simulink model "AccTarSel"  (R2018b)
settings: Solver=FixedStepDiscrete  StartTime=0.0  StopTime=inf  FixedStep=0.01  RelTol=1e-3
PostLoadFcn:
  | if any(exist('dsrtsu_mdlpostloadfcn', 'file') ~= 0), dsrtsu_mdlpostloadfcn('Execute', bdroot); end
values from neighbouring files (symbols this model uses):
  P_adtMaxBDC = 1.0    [AccTarSel.sldd]
  P_aFOCApproachIntpAcitve = -0.6    [AccTarSel.sldd]
  P_aFOCApproachIntpEnsure = -1.8    [AccTarSel.sldd]
  P_CutInEnable = 1.0    [AccTarSel.sldd]
  P_dAimMin = 4.5    [AccTarSel.sldd]
  P_dAimMinAVP = 1.5    [AccTarSel.sldd]
  P_dObjDrvOffMax = 5.0    [AccTarSel.sldd]
  P_dObjDrvOffMin = 3.0    [AccTarSel.sldd]
  P_dObjLowHystDecToStop = 4.5    [AccTarSel.sldd]
  P_dObjLowHystDecToStopAVP = 1.5    [AccTarSel.sldd]
  P_dObjUpperHystDecToStop = 5.0    [AccTarSel.sldd]
  P_dResMax = 5.0    [AccTarSel.sldd]
  P_dStandStill = 3.0    [AccTarSel.sldd]
  P_dStandStillMin = 2.0    [AccTarSel.sldd]
  P_dvarYMax4PO = 1.0    [AccTarSel.sldd]
  P_dyCutInThres = 3.6    [AccTarSel.sldd]
  P_facBDCInit = 0.7    [AccTarSel.sldd]
  P_facBDCIterCalc = 0.8    [AccTarSel.sldd]
  P_facFOCNegDiff = 0.3    [AccTarSel.sldd]
  P_facFOCPosDiff = 0.2    [AccTarSel.sldd]
  P_kapHystThres = 0.0005    [AccTarSel.sldd]
  P_PlausIntegDisable = 0.0    [AccTarSel.sldd]
  P_plausMin4PO = 0.5    [AccTarSel.sldd]
  P_probExistMin4PO = 0.8    [AccTarSel.sldd]
  P_StandObjEnable = 0.0    [AccTarSel.sldd]
  P_tAxTrackNegLower = 0.3    [AccTarSel.sldd]
  P_tAxTrackNegUpper = 0.6    [AccTarSel.sldd]
  P_tAxTrackPosLower = 1.0    [AccTarSel.sldd]
  P_tAxTrackPosUpper = 2.0    [AccTarSel.sldd]
  P_tBDCStartFilt = 0.2    [AccTarSel.sldd]
  P_tCSC = 3.5    [AccTarSel.sldd]
  P_tCurvFilt = 0.2    [AccTarSel.sldd]
  P_tCutInFilt = 0.5    [AccTarSel.sldd]
  P_tFiltAxAbsPONegFast = 0.1    [AccTarSel.sldd]
  P_tFiltAxAbsPONegSlow = 0.4    [AccTarSel.sldd]
  P_tFiltAxAbsPOPosFast = 1.2    [AccTarSel.sldd]
  P_tFiltAxAbsPOPosSlow = 2.0    [AccTarSel.sldd]
  P_tFiltAxAbsPOStand = 2.0    [AccTarSel.sldd]
  P_tFiltDAim = 0.1    [AccTarSel.sldd]
  P_tFiltDsd = 0.1    [AccTarSel.sldd]
  P_tFiltSpdLim = 3.0    [AccTarSel.sldd]
  P_tFiltVxAxPOFast = 0.15    [AccTarSel.sldd]
  P_tFiltVxAxPOSlow = 0.25    [AccTarSel.sldd]
  P_tFOCStatAccelFast = 4.0    [AccTarSel.sldd]
  P_tFOCStatAccelSlow = 3.5    [AccTarSel.sldd]
  P_tFOCStatDecelFast = 4.0    [AccTarSel.sldd]
  P_tFOCStatDecelSlow = 3.2    [AccTarSel.sldd]
  P_tMinDrvPhase = 2.0    [AccTarSel.sldd]
  P_tPredObjLeav = 1.2    [AccTarSel.sldd]
  P_tRollingFilt = 0.5    [AccTarSel.sldd]
  P_tRollingFinFilt = 1.0    [AccTarSel.sldd]
  P_tSSCNeg = 4.5    [AccTarSel.sldd]
  P_tSSCPos = 5.5    [AccTarSel.sldd]
  P_tToStop = 5.0    [AccTarSel.sldd]
  P_tToStopInBDC = 6.0    [AccTarSel.sldd]
  P_tToStopTrig = 4.0    [AccTarSel.sldd]
  P_vEgoDecToStop = 3.0    [AccTarSel.sldd]
  P_vEgoLowBDC = 4.0    [AccTarSel.sldd]
  P_vFOCNegDiff = 4.0    [AccTarSel.sldd]
  P_vFOCPosDiff = 5.0    [AccTarSel.sldd]
  P_vFOCStationaryFast = 15.0    [AccTarSel.sldd]
  P_vFOCStationarySlow = 5.0    [AccTarSel.sldd]
  P_vObjDrvOff = 0.5    [AccTarSel.sldd]
  P_vObjLowHystDecToStop = 0.5    [AccTarSel.sldd]
  P_vObjNoStop = 1.0    [AccTarSel.sldd]
  P_vObjReCalc = 1.0    [AccTarSel.sldd]
  P_vObjStop = 0.3    [AccTarSel.sldd]
  P_vObjUpperHystDecToStop = 0.8    [AccTarSel.sldd]
  P_vStandStill = 0.3    [AccTarSel.sldd]
  P_vStandStillHyst = 0.3    [AccTarSel.sldd]
  P_vyCutInThres = 0.5    [AccTarSel.sldd]
libraries: simulink x21, LPFilter x12
(part 2 of 11)

== system AccTarSel/EgoCourseFusion ==
  egoInfo : Inport
  SYS_Info_st : Inport  Port=2
  Bus Creator : BusCreator  Inputs=4  OutDataTypeStr=Bus: TRAJ_LANE_ST
  Bus Selector : BusSelector  OutputSignals=Curvature
  Bus Selector1 : BusSelector  OutputSignals=dT
  Constant2 : Constant  Value=0.5  OutDataTypeStr=single
  Constant3 : Constant  Value=0  OutDataTypeStr=single
  Constant4 : Constant  Value=0  OutDataTypeStr=single
  Constant5 : Constant  Value=0  OutDataTypeStr=single
  CurvatureFilt : Subsystem
  Multiply : Product
  egoTrajLane_st : Outport
  wires:
  Bus Creator/1 -> egoTrajLane_st/1  "egoTrajLane_st"
  CurvatureFilt/1(kapTrajFilt) -> Multiply/1  "kapTrajFilt"
  Constant2/1 -> Multiply/2
  Constant4/1 -> Bus Creator/3  "c"
  Constant3/1 -> Bus Creator/1  "a"
  Multiply/1 -> Bus Creator/2  "b"
  Constant5/1 -> Bus Creator/4  "d"
  egoInfo/1 -> Bus Selector/1
  Bus Selector/1 -> CurvatureFilt/1(In1)  "<Curvature>"
  SYS_Info_st/1 -> Bus Selector1/1
  Bus Selector1/1 -> CurvatureFilt/2(In2)  "<dT>"

== system AccTarSel/ObjAdapter ==
  FusObjIn : Inport
  egoInfo : Inport  Port=2
  Bus Creator : BusCreator  Inputs=2  OutDataTypeStr=Bus: FUS_OBJDATA_ST  NonVirtualBus=on
  Bus Selector : BusSelector  OutputSignals=objects
  Constant : Constant  Value=0  OutDataTypeStr=double
  For Each Subsystem : Subsystem  TreatAsAtomicUnit=on
  FusObjOut : Outport  OutDataTypeStr=Bus: FUS_OBJDATA_ST
  wires:
  FusObjIn/1 -> Bus Selector/1
  Bus Selector/1 -> For Each Subsystem/1(In1)  "<objects>"
  Bus Creator/1 -> FusObjOut/1
  For Each Subsystem/1(Out1) -> Bus Creator/2  "objdata_st"
  Constant/1 -> Bus Creator/1  "timeStamp"
  egoInfo/1 -> For Each Subsystem/2(In2)

== system AccTarSel/ObjRadarAdapter ==
  In1 : Inport
  Bus Creator : BusCreator  Inputs=2  OutDataTypeStr=Bus: FUS_OBJDATA_ST  NonVirtualBus=on
      settings: InheritFromInputs=off
  Bus Selector : BusSelector  OutputSignals=x50_20_Obj_00,x51_21_Obj_01,x52_22_Obj_02,x53_23_Obj_03,x54_24_Obj_04,x55_25_Obj_05,x56_26_Obj_06,x57_27_Obj_07,x58_28_Obj_08,x59_29_Obj_09,x5A_2A_Obj_10,x5B_2B_Obj_11,x5C_2C_Obj_12,x5D_2D_Obj_13,x5E_2E_Obj_14,x5F_2F_Obj_15,x60_30_Obj_16,x61_31_Obj_17,x62_32_Obj_18,x63_33_Obj_19,x64_34_Obj_20,x65_35_Obj_21,x66_36_Obj_22,x67_37_Obj_23,x68_38_Obj_24,x69_39_Obj_25,x6A_3A_Obj_26,x6B_3B_Obj_27,x6C_3C_Obj_28,x6D_3D_Obj_29,x6E_3E_Obj_30,x6F_3F_Obj_31,x70_40_Obj_32,x71_41_Obj_33,x72_42_Obj_34,x73_43_Obj_35,x74_44_Obj_36,x75_45_Obj_37,x76_46_Obj_38,x77_47_Obj_39
  Constant : Constant  Value=0  OutDataTypeStr=double
  For Each Subsystem : Subsystem  TreatAsAtomicUnit=on
  Vector Concatenate : Concatenate  NumInputs=40
  RadarObjOut : Outport  OutDataTypeStr=Bus: FUS_OBJDATA_ST
  wires:
  In1/1 -> Bus Selector/1
  Bus Selector/1 -> Vector Concatenate/1  "<x50_20_Obj_00>"
  Bus Selector/2 -> Vector Concatenate/2  "<x51_21_Obj_01>"
  Bus Selector/3 -> Vector Concatenate/3  "<x52_22_Obj_02>"
  Bus Selector/4 -> Vector Concatenate/4  "<x53_23_Obj_03>"
  Bus Selector/5 -> Vector Concatenate/5  "<x54_24_Obj_04>"
  Bus Selector/6 -> Vector Concatenate/6  "<x55_25_Obj_05>"
  Bus Selector/7 -> Vector Concatenate/7  "<x56_26_Obj_06>"
  Bus Selector/8 -> Vector Concatenate/8  "<x57_27_Obj_07>"
  Bus Selector/9 -> Vector Concatenate/9  "<x58_28_Obj_08>"
  Bus Selector/10 -> Vector Concatenate/10  "<x59_29_Obj_09>"
  Bus Selector/11 -> Vector Concatenate/11  "<x5A_2A_Obj_10>"
  Bus Selector/12 -> Vector Concatenate/12  "<x5B_2B_Obj_11>"
  Bus Selector/13 -> Vector Concatenate/13  "<x5C_2C_Obj_12>"
  Bus Selector/14 -> Vector Concatenate/14  "<x5D_2D_Obj_13>"
  Bus Selector/15 -> Vector Concatenate/15  "<x5E_2E_Obj_14>"
  Bus Selector/16 -> Vector Concatenate/16  "<x5F_2F_Obj_15>"
  Bus Selector/17 -> Vector Concatenate/17  "<x60_30_Obj_16>"
  Bus Selector/18 -> Vector Concatenate/18  "<x61_31_Obj_17>"
  Bus Selector/19 -> Vector Concatenate/19  "<x62_32_Obj_18>"
  Bus Selector/20 -> Vector Concatenate/20  "<x63_33_Obj_19>"
  Bus Selector/21 -> Vector Concatenate/21  "<x64_34_Obj_20>"
  Bus Selector/22 -> Vector Concatenate/22  "<x65_35_Obj_21>"
  Bus Selector/23 -> Vector Concatenate/23  "<x66_36_Obj_22>"
  Bus Selector/24 -> Vector Concatenate/24  "<x67_37_Obj_23>"
  Bus Selector/25 -> Vector Concatenate/25  "<x68_38_Obj_24>"
  Bus Selector/26 -> Vector Concatenate/26  "<x69_39_Obj_25>"
  Bus Selector/27 -> Vector Concatenate/27  "<x6A_3A_Obj_26>"
  Bus Selector/28 -> Vector Concatenate/28  "<x6B_3B_Obj_27>"
  Bus Selector/29 -> Vector Concatenate/29  "<x6C_3C_Obj_28>"
  Bus Selector/30 -> Vector Concatenate/30  "<x6D_3D_Obj_29>"
  Bus Selector/31 -> Vector Concatenate/31  "<x6E_3E_Obj_30>"
  Bus Selector/32 -> Vector Concatenate/32  "<x6F_3F_Obj_31>"
  Bus Selector/33 -> Vector Concatenate/33  "<x70_40_Obj_32>"
  Bus Selector/34 -> Vector Concatenate/34  "<x71_41_Obj_33>"
  Bus Selector/35 -> Vector Concatenate/35  "<x72_42_Obj_34>"
  Bus Selector/36 -> Vector Concatenate/36  "<x73_43_Obj_35>"
  Bus Selector/37 -> Vector Concatenate/37  "<x74_44_Obj_36>"
  Bus Selector/38 -> Vector Concatenate/38  "<x75_45_Obj_37>"
  Bus Selector/39 -> Vector Concatenate/39  "<x76_46_Obj_38>"
  Bus Selector/40 -> Vector Concatenate/40  "<x77_47_Obj_39>"
  Vector Concatenate/1 -> For Each Subsystem/1(In1)
  For Each Subsystem/1(Out1) -> Bus Creator/2  "objdata_st"
  Bus Creator/1 -> RadarObjOut/1
  Constant/1 -> Bus Creator/1  "timeStamp"

== system AccTarSel/RTI Data ==
  RTI Data Store : Subsystem  Tag="struct('private',struct('version',struct('dsVer',uint32(2),'dsVerCreation',uint32(2),'RTI',struct('ver','7.12','type','RTI1401')),'access',struct('type','Model','isPerm',1,'created',['19-Nov-2020 15:49:14'],'modified',['12-Mar-2021 13:34:18'],'location','')),'public',struct('main',struct('data',[]),'sub',struct('name',{{'AccTarSel'}},'data',{{struct('TH',struct('thTaskInfo',struct('taskType',{'TIMER','HWINT','TMRINT','SWINT','GLINT'},'tasksNumOf',{1,0,0,0,0},'srcIds',{{'TIMERA'},{},{},{},{}},'taskNames',{{['Timer Task 1']},{},{},{},{}})),'th_tc',struct('dataType','TASK','taskGroupId','','taskGroupList',{{}},'taskSchedulingPolicy','FCFS','taskType','TIMER','blkh',-1,'srcId','TIMERA','srcSgnName',['Timer A interrupt'],'srcCpuName','','taskName',['Timer Task 1  [0.005] s'],'taskNameDisplayExt','','smplTime',0.005,'smplTimeOffs',0,'hasFixedPriority',0,'priority',1,'hasFixedOvc',0,'ovcType',1,'ovcMax',1),'tc_th',struct('dataType','TASK','taskGroupId','','taskGroupList',{{}},'taskSchedulingPolicy','FCFS','taskType','TIMER','blkh',-1,'srcId','TIMERA','srcSgnName',['Timer A interrupt'],'srcCpuName','','taskName',['Timer Task 1  [0.005] s'],'taskNameDisplayExt','','smplTime',0.005,'smplTimeOffs',0,'hasFixedPriority',0,'priority',1,'hasFixedOvc',0,'ovcType',1,'ovcMax',1))}})))"  mask(RTI_DATA_STORE){}
      mask help:
      | RTI Data Store Block. This block is used by RTI to store internal model dependent data. Deleting this block will result in data loss.
      |
      | NEVER DELETE, COPY, OR MODIFY THIS BLOCK!
      mask Help:
      | RTI Data Store Block. This block is used by RTI to store internal model dependent data. Deleting this block will result in data loss.
      | 
      | NEVER DELETE, COPY, OR MODIFY THIS BLOCK!
      mask Display: text(0.5, 0.5, ' ', 'HorizontalAlignment', 'center');

== system AccTarSel/Subsystem ==
  In1 : Inport
  In2 : Inport  Port=2
  Bus Creator : BusCreator  Inputs=2  OutDataTypeStr=Bus: FUS_OBJDATA_ST  NonVirtualBus=on
  Bus Selector : BusSelector  OutputSignals=timeStamp,objdata_st
  Bus Selector1 : BusSelector  OutputSignals=objdata_st
  Vector Concatenate : Concatenate  ConcatenateDimension=2
  Out1 : Outport
  wires:
  In1/1 -> Bus Selector/1
  In2/1 -> Bus Selector1/1
  Bus Selector1/1 -> Vector Concatenate/2  "<objdata_st>"
  Bus Selector/2 -> Vector Concatenate/1  "<objdata_st>"
  Bus Selector/1 -> Bus Creator/1  "<timeStamp>"
  Vector Concatenate/1 -> Bus Creator/2  "objdata_st"
  Bus Creator/1 -> Out1/1

== system AccTarSel/Subsystem1 ==
  objInfo : Inport
  egoInfo : Inport  Port=2
  AND2 : Logic  AllPortsSameDT=off  OutDataTypeStr=boolean
  AND3 : Logic  Operator=OR  AllPortsSameDT=off  OutDataTypeStr=boolean
  Add : Sum
  Bus Selector : BusSelector  OutputSignals=Valid,dx,vx
  Bus Selector1 : BusSelector  OutputSignals=vRef
  Constant : Constant  OutDataTypeStr=boolean
  Constant1 : Constant  Value=0  OutDataTypeStr=int32
  If : If  IfExpression=u1 == 1
  If Action Subsystem : Subsystem  TreatAsAtomicUnit=on
  If Action Subsystem1 : Subsystem  TreatAsAtomicUnit=on
  Merge : Merge
  P_dObjDrvOffMax : Constant  Value=P_dObjDrvOffMax
  P_dObjDrvOffMin : Constant  Value=P_dObjDrvOffMin
  P_vObjDrvOff : Constant  Value=P_vObjDrvOff
  Relational Operator6 : RelationalOperator  Operator=>  OutDataTypeStr=boolean  RndMeth=Simplest
  Relational Operator7 : RelationalOperator  Operator=>  OutDataTypeStr=boolean  RndMeth=Simplest
  Relational Operator8 : RelationalOperator  Operator=>  OutDataTypeStr=boolean  RndMeth=Simplest
  Selector1 : Selector  IndexMode=Zero-based  InputPortWidth=6  IndexOptions=Index vector (port)  Indices=[1 3]  OutputSizes=1
  DrvOffEnable : Outport
  wires:
  AND2/1 -> AND3/2
  Relational Operator8/1 -> AND2/2
  Add/1 -> Relational Operator8/1  "vAbsObj"
  P_dObjDrvOffMin/1 -> Relational Operator7/2
  Relational Operator7/1 -> AND2/1
  Relational Operator6/1 -> AND3/1
  P_vObjDrvOff/1 -> Relational Operator8/2
  P_dObjDrvOffMax/1 -> Relational Operator6/2
  Bus Selector/1 -> If/1  "<Valid>"
  egoInfo/1 -> Bus Selector1/1
  Bus Selector1/1 -> Add/2  "<vRef>"
  Bus Selector/3 -> Add/1  "<vx>"
  Bus Selector/2 -> Relational Operator6/1, Relational Operator7/1  "<dx>"
  AND3/1 -> If Action Subsystem/1(In1)
  Constant/1 -> If Action Subsystem1/1(In1)
  If/1 -> If Action Subsystem/Action
  If/2 -> If Action Subsystem1/Action
  If Action Subsystem/1(Out1) -> Merge/1
  If Action Subsystem1/1(Out1) -> Merge/2
  Merge/1 -> DrvOffEnable/1  "DrvOffEnable"
  objInfo/1 -> Selector1/1
  Constant1/1 -> Selector1/2
  Selector1/1 -> Bus Selector/1

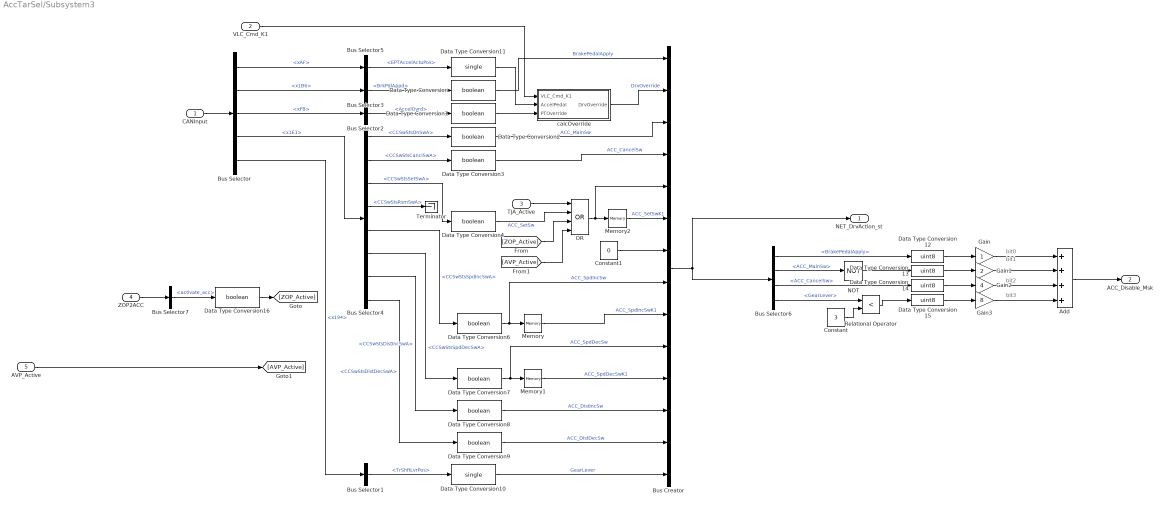
== system AccTarSel/Subsystem3 ==
  note: bit0
  note: bit1
  note: bit2
  note: bit3
  CANInput : Inport
  VLC_Cmd_K1 : Inport  Port=2
  TJA_Active : Inport  Port=3
  ZOP2ACC : Inport  Port=4
  AVP_Active : Inport  Port=5
  Add : Sum  Inputs=++++  AccumDataTypeStr=uint16
  Bus Creator : BusCreator  Inputs=14  OutDataTypeStr=Bus: NET_DRVACTION_ST  NonVirtualBus=on
      settings: InheritFromInputs=off
  Bus Selector : BusSelector  OutputSignals=xAF,x1B6,xFB,x1E1,x194
  Bus Selector1 : BusSelector  OutputSignals=TrShftLvrPos
  Bus Selector2 : BusSelector  OutputSignals=AccelOvrd
  Bus Selector3 : BusSelector  OutputSignals=BrkPdlAppd
  Bus Selector4 : BusSelector  OutputSignals=CCSwStsOnSwA,CCSwStsCanclSwA,CCSwStsSetSwA,CCSwStsRsmSwA,CCSwStsSpdIncSwA,CCSwStsSpdDecSwA,CCSwStsDistIncSwA,CCSwStsDistDecSwA
  Bus Selector5 : BusSelector  OutputSignals=EPTAccelActuPos
  Bus Selector6 : BusSelector  OutputSignals=BrakePedalApply,ACC_MainSw,ACC_CancelSw,GearLever
  Bus Selector7 : BusSelector  OutputSignals=activate_acc
  Constant : Constant  Value=3  OutDataTypeStr=single
  Constant1 : Constant  Value=0  OutDataTypeStr=boolean
  Data Type Conversion{,1..4,6..9,16} (10 alike) : DataTypeConversion  OutDataTypeStr=boolean
  Data Type Conversion10 : DataTypeConversion  OutDataTypeStr=single
  Data Type Conversion11 : DataTypeConversion  OutDataTypeStr=single
  Data Type Conversion{12..15} (4 alike) : DataTypeConversion  OutDataTypeStr=uint8
  Gain : Gain  OutDataTypeStr=uint16
  Gain1 : Gain  Gain=2  OutDataTypeStr=uint16
  Gain2 : Gain  Gain=4  OutDataTypeStr=uint16
  Gain3 : Gain  Gain=8  OutDataTypeStr=uint16
  Memory : Memory
  Memory1 : Memory
  Memory2 : Memory
  NOT : Logic  Operator=NOT  AllPortsSameDT=off  OutDataTypeStr=boolean
  OR : Logic  Operator=OR  Inputs=4  AllPortsSameDT=off  OutDataTypeStr=boolean
  Relational Operator : RelationalOperator  Operator=<  OutDataTypeStr=boolean  RndMeth=Simplest
  Terminator : Terminator
  calcOverride : Subsystem
  NET_DrvAction_st : Outport  OutDataTypeStr=Bus: NET_DRVACTION_ST
  ACC_Disable_Msk : Outport  Port=2
  wires:
  CANInput/1 -> Bus Selector/1
  Bus Selector/5 -> Bus Selector1/1  "<x194>"
  Bus Selector/3 -> Bus Selector2/1  "<xFB>"
  Bus Selector/2 -> Bus Selector3/1  "<x1B6>"
  Bus Selector/4 -> Bus Selector4/1  "<x1E1>"
  Bus Selector3/1 -> Data Type Conversion/1  "<BrkPdlAppd>"
  Data Type Conversion/1 -> Bus Creator/1  "BrakePedalApply"
  Bus Selector2/1 -> Data Type Conversion1/1  "<AccelOvrd>"
  Bus Selector4/1 -> Data Type Conversion2/1  "<CCSwStsOnSwA>"
  Bus Selector4/2 -> Data Type Conversion3/1  "<CCSwStsCanclSwA>"
  Bus Selector4/3 -> Data Type Conversion4/1  "<CCSwStsSetSwA>"
  Bus Selector4/4 -> Terminator/1  "<CCSwStsRsmSwA>"
  Bus Selector4/5 -> Data Type Conversion6/1  "<CCSwStsSpdIncSwA>"
  Bus Selector4/6 -> Data Type Conversion7/1  "<CCSwStsSpdDecSwA>"
  Data Type Conversion6/1 -> Bus Creator/8, Memory/1  "ACC_SpdIncSw"
  Memory/1 -> Bus Creator/9  "ACC_SpdIncSwK1"
  Data Type Conversion7/1 -> Bus Creator/10, Memory1/1  "ACC_SpdDecSw"
  Memory1/1 -> Bus Creator/11  "ACC_SpdDecSwK1"
  Data Type Conversion8/1 -> Bus Creator/12  "ACC_DistIncSw"
  Bus Selector4/7 -> Data Type Conversion8/1  "<CCSwStsDistIncSwA>"
  Data Type Conversion9/1 -> Bus Creator/13  "ACC_DistDecSw"
  Bus Selector4/8 -> Data Type Conversion9/1  "<CCSwStsDistDecSwA>"
  Data Type Conversion2/1 -> Bus Creator/3  "ACC_MainSw"
  Data Type Conversion3/1 -> Bus Creator/4  "ACC_CancelSw"
  Bus Creator/1 -> NET_DrvAction_st/1, Bus Selector6/1
  Data Type Conversion10/1 -> Bus Creator/14  "GearLever"
  Bus Selector1/1 -> Data Type Conversion10/1  "<TrShftLvrPos>"
  Bus Selector/1 -> Bus Selector5/1  "<xAF>"
  Bus Selector5/1 -> Data Type Conversion11/1  "<EPTAccelActuPos>"
  calcOverride/1(DrvOverride) -> Bus Creator/2  "DrvOverride"
  VLC_Cmd_K1/1 -> calcOverride/1(VLC_Cmd_K1)
  Data Type Conversion11/1 -> calcOverride/2(AccelPedal)
  Data Type Conversion1/1 -> calcOverride/3(PTOverride)
  Memory2/1 -> Bus Creator/6  "ACC_SetSwK1"
  Bus Selector6/1 -> Data Type Conversion12/1  "<BrakePedalApply>"
  Bus Selector6/3 -> Data Type Conversion14/1  "<ACC_CancelSw>"
  Bus Selector6/2 -> NOT/1  "<ACC_MainSw>"
  NOT/1 -> Data Type Conversion13/1
  Bus Selector6/4 -> Relational Operator/1  "<GearLever>"
  Constant/1 -> Relational Operator/2
  Relational Operator/1 -> Data Type Conversion15/1
  Data Type Conversion12/1 -> Gain/1
  Data Type Conversion13/1 -> Gain1/1
  Data Type Conversion14/1 -> Gain2/1
  Data Type Conversion15/1 -> Gain3/1
  Gain/1 -> Add/1
  Gain1/1 -> Add/2
  Gain2/1 -> Add/3
  Gain3/1 -> Add/4
  Add/1 -> ACC_Disable_Msk/1
  TJA_Active/1 -> OR/1
  Data Type Conversion4/1 -> OR/2  "ACC_SetSw"
  OR/1 -> Bus Creator/5, Memory2/1
  Constant1/1 -> Bus Creator/7
  ZOP2ACC/1 -> Bus Selector7/1
  Bus Selector7/1 -> Data Type Conversion16/1  "<activate_acc>"
  Data Type Conversion16/1 -> [ZOP_Active]
  [ZOP_Active] -> OR/3
  AVP_Active/1 -> [AVP_Active]
  [AVP_Active] -> OR/4

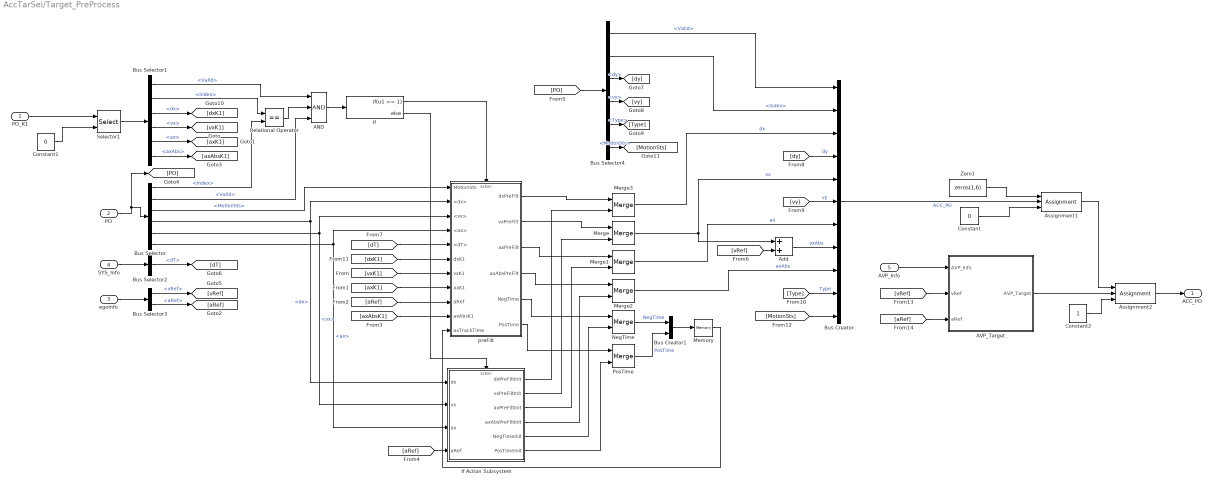
== system AccTarSel/Target_PreProcess ==
  PO_K1 : Inport
  PO : Inport  Port=2
  egoInfo : Inport  Port=3
  SYS_Info : Inport  Port=4
  AVP_Info : Inport  Port=5
  AND : Logic  Inputs=3  AllPortsSameDT=off  OutDataTypeStr=boolean
  AVP_Target : Subsystem
  Add : Sum
  Assignment1 : Assignment  IndexMode=Zero-based  DiagnosticForDimensions=Warning  IndexOptions=Index vector (port)  Indices=1  OutputSizes=1
  Assignment2 : Assignment  IndexMode=Zero-based  DiagnosticForDimensions=Warning  IndexOptions=Index vector (port)  Indices=1  OutputSizes=1
  Bus Creator : BusCreator  Inputs=11  OutDataTypeStr=Bus: ATS_PO_ST  NonVirtualBus=on
      settings: InheritFromInputs=off
  Bus Creator1 : BusCreator  Inputs=2
  Bus Selector : BusSelector  OutputSignals=Index,Valid,MotionSts,dx,vx,ax
  Bus Selector1 : BusSelector  OutputSignals=Valid,Index,dx,vx,ax,axAbs
  Bus Selector2 : BusSelector  OutputSignals=dT
  Bus Selector3 : BusSelector  OutputSignals=vRef,aRef
  Bus Selector4 : BusSelector  OutputSignals=Valid,Index,dy,vy,Type,MotionSts
  Constant : Constant  Value=0  OutDataTypeStr=int32
  Constant1 : Constant  Value=0  OutDataTypeStr=int32
  Constant2 : Constant  OutDataTypeStr=int32
  If : If  IfExpression=u1 == 1
  If Action Subsystem : Subsystem  TreatAsAtomicUnit=on
  Memory : Memory
  Merge{,1..3} (4 alike) : Merge
  NegTime : Merge
  PosTime : Merge
  Relational Operator : RelationalOperator  Operator===  OutDataTypeStr=boolean  RndMeth=Simplest
  Selector1 : Selector  IndexMode=Zero-based  InputPortWidth=6  IndexOptions=Index vector (port)  Indices=[1 3]  OutputSizes=1
  Zero1 : Constant  Value=zeros(1,6)  OutDataTypeStr=Bus: ATS_PO_ST
  preFilt : Subsystem
  ACC_PO : Outport  OutDataTypeStr=Bus: ATS_PO_ST
  wires:
  PO/1 -> [PO], Bus Selector/1
  Bus Selector1/1 -> AND/1  "<Valid>"
  Bus Selector1/2 -> Relational Operator/1  "<Index>"
  Bus Selector/1 -> Relational Operator/2  "<Index>"
  Relational Operator/1 -> AND/2
  Bus Selector/2 -> AND/3  "<Valid>"
  SYS_Info/1 -> Bus Selector2/1
  Bus Selector1/4 -> [vxK1]  "<vx>"
  Bus Selector1/5 -> [axK1]  "<ax>"
  AND/1 -> If/1
  Bus Selector/5 -> preFilt/3(<vx>), If Action Subsystem/2(vx)  "<vx>"
  Bus Selector/6 -> preFilt/4(<ax>), If Action Subsystem/3(ax)  "<ax>"
  [vxK1] -> preFilt/7(vxK1)
  [axK1] -> preFilt/8(axK1)
  If/1 -> preFilt/Action
  If/2 -> If Action Subsystem/Action
  preFilt/2(vxPreFilt) -> Merge/1
  If Action Subsystem/2(vxPreFiltInit) -> Merge/2
  preFilt/3(axPreFilt) -> Merge1/1
  If Action Subsystem/3(axPreFiltInit) -> Merge1/2
  egoInfo/1 -> Bus Selector3/1
  Bus Selector3/2 -> [aRef]  "<aRef>"
  [aRef] -> preFilt/9(aRef)
  Bus Selector1/6 -> [axAbsK1]  "<axAbs>"
  [axAbsK1] -> preFilt/10(axAbsK1)
  [aRef] -> If Action Subsystem/4(aRef)
  preFilt/4(axAbsPreFilt) -> Merge2/1
  If Action Subsystem/4(axAbsPreFiltInit) -> Merge2/2
  [PO] -> Bus Selector4/1
  Bus Selector4/1 -> Bus Creator/1  "<Valid>"
  Bus Selector4/2 -> Bus Creator/2  "<Index>"
  Merge/1 -> Bus Creator/5, Add/1  "vx"
  Merge1/1 -> Bus Creator/7  "ax"
  Merge2/1 -> Bus Creator/9  "axAbs"
  Bus Creator/1 -> Assignment1/2  "ACC_PO"
  Bus Selector3/1 -> [vRef]  "<vRef>"
  Add/1 -> Bus Creator/8  "vxAbs"
  [vRef] -> Add/2
  Bus Selector/4 -> preFilt/2(<dx>), If Action Subsystem/1(dx)  "<dx>"
  [dxK1] -> preFilt/6(dxK1)
  Bus Selector2/1 -> [dT]  "<dT>"
  [dT] -> preFilt/5(<dT>)
  preFilt/1(dxPreFilt) -> Merge3/1
  If Action Subsystem/1(dxPreFiltInit) -> Merge3/2
  Merge3/1 -> Bus Creator/3  "dx"
  Bus Selector4/3 -> [dy]  "<dy>"
  [dy] -> Bus Creator/4  "dy"
  Bus Selector4/4 -> [vy]  "<vy>"
  [vy] -> Bus Creator/6  "vy"
  Bus Selector4/5 -> [Type]  "<Type>"
  [Type] -> Bus Creator/10  "Type"
  Bus Selector1/3 -> [dxK1]  "<dx>"
  Bus Selector4/6 -> [MotionSts]  "<MotionSts>"
  [MotionSts] -> Bus Creator/11
  preFilt/5(NegTime) -> NegTime/1
  If Action Subsystem/5(NegTimeInit) -> NegTime/2
  preFilt/6(PosTime) -> PosTime/1
  If Action Subsystem/6(PosTimeInit) -> PosTime/2
  NegTime/1 -> Bus Creator1/1  "NegTime"
  PosTime/1 -> Bus Creator1/2  "PosTime"
  Bus Creator1/1 -> Memory/1
  Memory/1 -> preFilt/11(axTrackTime)
  Bus Selector/3 -> preFilt/1(MotionSts)  "<MotionSts>"
  Zero1/1 -> Assignment1/1
  Constant/1 -> Assignment1/3
  Assignment1/1 -> Assignment2/1
  PO_K1/1 -> Selector1/1
  Constant1/1 -> Selector1/2
  Selector1/1 -> Bus Selector1/1
  AVP_Info/1 -> AVP_Target/1(AVP_Info)
  [vRef] -> AVP_Target/2(vRef)
  [aRef] -> AVP_Target/3(aRef)
  AVP_Target/1(AVP_Target) -> Assignment2/2
  Constant2/1 -> Assignment2/3
  Assignment2/1 -> ACC_PO/1

== system AccTarSel/ZOP_ENABLE ==
  In1 : Inport
  Bus Selector : BusSelector  OutputSignals=activate_acc
  Data Type Conversion16 : DataTypeConversion  OutDataTypeStr=boolean
  ZOP_Enable : Outport
  wires:
  In1/1 -> Bus Selector/1
  Bus Selector/1 -> Data Type Conversion16/1  "<activate_acc>"
  Data Type Conversion16/1 -> ZOP_Enable/1
